simulink model "Receiver_UnderTest_Float"  (R2017b)
settings: Solver=FixedStepDiscrete  StartTime=0.0  StopTime=0.052263  RelTol=1e-3
InitFcn:
  | modelSettingsFloat
undefined symbols (not defined in the file or in its folder): crcDecodeLag, magnitude, numTrainingSamples, RadioSampleRate, samplesPerSymbol, VibertiTracebackLength, xPreambleSeq
libraries: simulink x15, hdlsllib x2, commdigbbndpm3 x2, commsource2 x1, commcrc2 x1, dspstat3 x1, dspsigops x1, commseqgen3 x1, commsequence2 x1, commcnvcod2 x1, commutil2 x1, commfilt2 x1
(part 1 of 2)
settings Model: DataTypeOverride=Off  MinMaxOverflowLogging=MinMaxAndOverflow  FPTRunName=NoOverride  Creator=tcollins  LastModifiedBy=tcollins
settings DataIOCC: SaveOutput=off  SaveTime=off
settings OptimizationCC: BlockReduction=off  ConditionallyExecuteInputs=off  DefaultParameterBehavior=Inlined
settings DebuggingCC: AlgebraicLoopMsg=error  SingleTaskRateTransMsg=error
settings HardwareCC: ProdBitPerPointer=32  ProdBitPerSizeT=32  ProdBitPerPtrDiffT=32  ProdLargestAtomicFloat=None  ProdIntDivRoundTo=Undefined  ProdEndianess=Unspecified  ProdWordSize=32  ProdHWDeviceType=ASIC/FPGA->ASIC/FPGA  ProdEqTarget=off
settings CodeAppCC: StateflowObjectComments=on
settings SimscapeCC: SimscapeNormalizeSystem=off

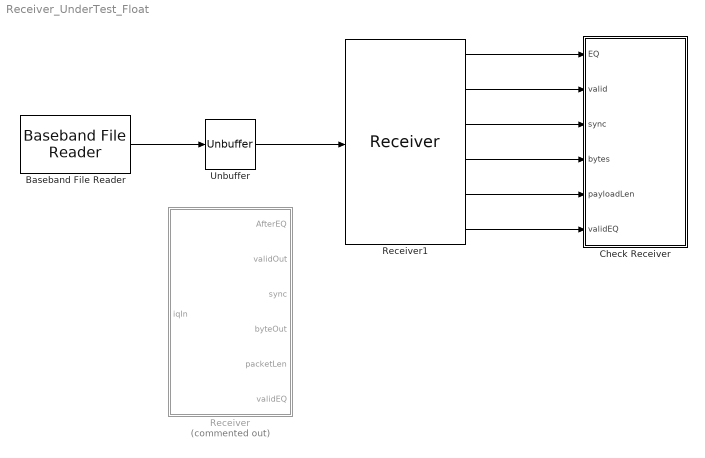
== system Receiver_UnderTest_Float ==
  Baseband File Reader : commsource2/Baseband File Reader  Filename=PlutoCaptureQPSK.bb  InheritSampleTimeFromFile=off  SampleTime=100000/(RadioSampleRate)  SamplesPerFrame=100000  CyclicRepetition=off  FileEndOutputPort=off  SimulateUsing=Interpreted execution
      settings: SourceProductName=Communications System Toolbox  SourceProductBaseCode=CM
  Check Receiver : Subsystem
  Receiver : Subsystem  Commented=on
  Receiver1 : RxFloatingPointLibrary/Receiver
  Unbuffer : Unbuffer
  wires:
  Baseband File Reader/1 -> Unbuffer/1
  Unbuffer/1 -> Receiver1/1
  Receiver1/1 -> Check Receiver/1(EQ)
  Receiver1/2 -> Check Receiver/2(valid)
  Receiver1/3 -> Check Receiver/3(sync)
  Receiver1/4 -> Check Receiver/4(bytes)
  Receiver1/5 -> Check Receiver/5(payloadLen)
  Receiver1/6 -> Check Receiver/6(validEQ)

== system Receiver_UnderTest_Float/Check Receiver ==
  EQ : Inport
  valid : Inport  Port=2
  sync : Inport  Port=3
  bytes : Inport  Port=4
  payloadLen : Inport  Port=5
  validEQ : Inport  Port=6
  Constellation Diagram : Subsystem
  DMA Capture : MATLAB Function  Commented=on  TreatAsAtomicUnit=on
  DMA Capture1 : MATLAB Function  TreatAsAtomicUnit=on
  To Workspace1 : ToWorkspace  VariableName=packetsFound  SaveFormat=Timeseries  SampleTime=-1
  To Workspace2 : ToWorkspace  VariableName=crcChecks  SaveFormat=Timeseries  SampleTime=-1
  To Workspace3 : ToWorkspace  VariableName=failures  SaveFormat=Timeseries  SampleTime=-1
  wires:
  EQ/1 -> Constellation Diagram/1(In1)
  sync/1 -> DMA Capture1/3(sync)
  validEQ/1 -> Constellation Diagram/Enable
  valid/1 -> DMA Capture1/2(validOut)
  bytes/1 -> DMA Capture1/1(bytes)
  payloadLen/1 -> DMA Capture1/4(payloadLen)
  DMA Capture1/2(crc) -> To Workspace2/1
  DMA Capture1/1(pf) -> To Workspace1/1
  DMA Capture1/3(failures) -> To Workspace3/1

== system Receiver_UnderTest_Float/Receiver ==
  iqIn : Inport
  CRC Check and DMA Pack : Subsystem
  Constellation Diagram : Subsystem
  Frame Recover : Subsystem
  Gardner Timing Recovery : Subsystem
  Raised Cosine Receive Filter : commfilt2/Raised Cosine Receive Filter  filtType=Square root  R=0.5  filtSpan=8  N=4  downFactor=1  downOffset=0  filterGain=1  RateOptions=Allow multirate processing  framing=Mute  checkCoeff=off  variableName=rcRxFilt  currentFiltSpan=8  D=(8)/2  inputOffset=0  sampMode=Mute  saveAsFlag=0  rateMode=Downsampling  checkGain=Normalized  launchFVT=on  roundingMode=Floor  overflowMode=off  coeffDataTypeStr=Inherit: Same word length as input  coeffMin=[]  coeffMax=[]  coeffLastDataTypeStr=Inherit: Same word length as input  accumDataTypeStr=Inherit: Same as product output  accumLastDataTypeStr=Inherit: Same as product output  outputDataTypeStr=Inherit: Same as accumulator  outputMin=[]  outputMax=[]  outputLastDataTypeStr=Inherit: Same as accumulator
  AfterEQ : Outport
  validOut : Outport  Port=2
  sync : Outport  Port=3
  byteOut : Outport  Port=4
  packetLen : Outport  Port=5
  validEQ : Outport  Port=6
  wires:
  Frame Recover/2(validOut) -> CRC Check and DMA Pack/1(validIn), validEQ/1
  CRC Check and DMA Pack/4(payloadLenOut) -> packetLen/1
  CRC Check and DMA Pack/3(sync) -> sync/1
  CRC Check and DMA Pack/1(byteOut) -> byteOut/1
  CRC Check and DMA Pack/2(validOut) -> validOut/1
  Frame Recover/6(packetLen) -> CRC Check and DMA Pack/5(payloadLen)
  Frame Recover/3(data) -> CRC Check and DMA Pack/2(bits)
  Frame Recover/5(frameEnd) -> CRC Check and DMA Pack/4(endCRC)
  Frame Recover/4(frameStart) -> CRC Check and DMA Pack/3(startData)
  Frame Recover/1(AfterEQ) -> AfterEQ/1
  iqIn/1 -> Raised Cosine Receive Filter/1
  Raised Cosine Receive Filter/1 -> Gardner Timing Recovery/1(dataIn)
  Gardner Timing Recovery/2(strobe) -> Frame Recover/Enable, Frame Recover/2(validIn), Constellation Diagram/Enable
  Gardner Timing Recovery/1(dataOut) -> Frame Recover/1(dataIn), Constellation Diagram/1(In1)

== system Receiver_UnderTest_Float/Check Receiver/Constellation Diagram ==
  In1 : Inport
  Enable : EnablePort
  Terminator : Terminator
  wires:
  In1/1 -> Terminator/1

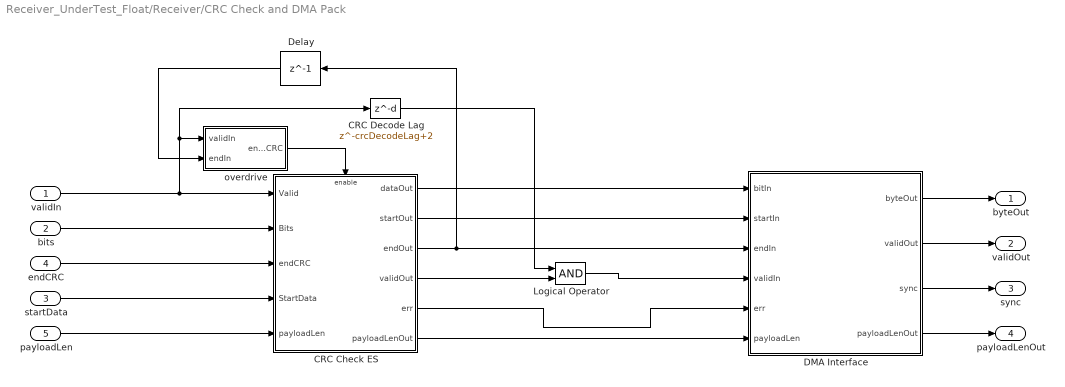
== system Receiver_UnderTest_Float/Receiver/CRC Check and DMA Pack ==
  validIn : Inport
  bits : Inport  Port=2
  startData : Inport  Port=3
  endCRC : Inport  Port=4
  payloadLen : Inport  Port=5
  CRC Check ES : Subsystem
  CRC Decode Lag : Delay  DelayLength=crcDecodeLag+2
  DMA Interface : Subsystem
  Delay : Delay  DelayLength=1
  Logical Operator : Logic  AllPortsSameDT=off  OutDataTypeStr=boolean
  overdrive : MATLAB Function  TreatAsAtomicUnit=on
  byteOut : Outport
  validOut : Outport  Port=2
  sync : Outport  Port=3
  payloadLenOut : Outport  Port=4
  wires:
  overdrive/1(enableCRC) -> CRC Check ES/Enable
  DMA Interface/4(payloadLenOut) -> payloadLenOut/1
  Delay/1 -> overdrive/2(endIn)
  validIn/1 -> overdrive/1(validIn), CRC Decode Lag/1, CRC Check ES/1(Valid)
  CRC Check ES/4(validOut) -> Logical Operator/2
  CRC Decode Lag/1 -> Logical Operator/1
  CRC Check ES/6(payloadLenOut) -> DMA Interface/6(payloadLen)
  CRC Check ES/5(err) -> DMA Interface/5(err)
  Logical Operator/1 -> DMA Interface/4(validIn)
  CRC Check ES/3(endOut) -> Delay/1, DMA Interface/3(endIn)
  CRC Check ES/2(startOut) -> DMA Interface/2(startIn)
  CRC Check ES/1(dataOut) -> DMA Interface/1(bitIn)
  endCRC/1 -> CRC Check ES/3(endCRC)
  startData/1 -> CRC Check ES/4(StartData)
  payloadLen/1 -> CRC Check ES/5(payloadLen)
  DMA Interface/3(sync) -> sync/1
  bits/1 -> CRC Check ES/2(Bits)
  DMA Interface/1(byteOut) -> byteOut/1
  DMA Interface/2(validOut) -> validOut/1

== system Receiver_UnderTest_Float/Receiver/Constellation Diagram ==
  In1 : Inport
  Enable : EnablePort
  wires:
  In1/1 -> ?

== system Receiver_UnderTest_Float/Receiver/Frame Recover ==
  dataIn : Inport
  validIn : Inport  Port=2
  Enable : EnablePort
  Barker Locate : Subsystem  mask{Threshold=1.4}
  Enable Equalizer and Packet Decode (Latch) : MATLAB Function  TreatAsAtomicUnit=on
  Equalization and Demodulation : Subsystem
  Frequency Recovery : Subsystem
  AfterEQ : Outport
  validOut : Outport  Port=2  OutputWhenDisabled=reset  InitialOutput=0
  data : Outport  Port=3
  frameStart : Outport  Port=4
  frameEnd : Outport  Port=5
  packetLen : Outport  Port=6
  wires:
  Equalization and Demodulation/6(frameStart) -> frameStart/1
  Equalization and Demodulation/4(dataOut) -> data/1
  Equalization and Demodulation/1(AfterEQ) -> AfterEQ/1
  Equalization and Demodulation/2(validOut) -> validOut/1
  Equalization and Demodulation/3(crcEnd) -> frameEnd/1
  Enable Equalizer and Packet Decode (Latch)/1(enable) -> Equalization and Demodulation/Enable
  Barker Locate/2(Signal) -> Equalization and Demodulation/2(Data)
  Barker Locate/3(enableOut) -> Enable Equalizer and Packet Decode (Latch)/2(validIn)
  Barker Locate/1(Detector) -> Equalization and Demodulation/1(Trigger), Enable Equalizer and Packet Decode (Latch)/1(start)
  Equalization and Demodulation/5(packLen) -> packetLen/1
  Frequency Recovery/1(dataOut) -> Barker Locate/1(In1)
  Frequency Recovery/2(validOut) -> Barker Locate/2(enableIn)
  dataIn/1 -> Frequency Recovery/1(dataIn)
  validIn/1 -> Frequency Recovery/2(validIn)

== system Receiver_UnderTest_Float/Receiver/Gardner Timing Recovery ==
  dataIn : Inport
  Delay : Delay  DelayLength=1
  Delay1 : Delay  DelayLength=1
  Gardner TED Blocks : Subsystem
  InterpControl_Blocks1 : Subsystem
  Interpolator : Subsystem
  LoopFilter : Subsystem  mask{zeta=sqrt(2), BnTs=0.01, Kp=2.7}
      mask prompts: zeta "DampingFactor"; BnTs "NormalizedLoopBandwidth"; Kp "DetectionGain"
      mask init:
      | K0 = -1;
      | SPS = 4;
      | theta = BnTs/SPS/(zeta + 0.25/zeta);
      | d  = (1 + 2*zeta*theta + theta^2) * K0 * Kp;
      | ProportionalGain = (4*zeta*theta) /d;
      | IntegratorGain   = (4*theta*theta)/d;
  dataOut : Outport  InitialOutput=0
  strobe : Outport  Port=2  InitialOutput=false
  wires:
  dataIn/1 -> Interpolator/1(In1)
  LoopFilter/1(v) -> InterpControl_Blocks1/1(e)
  InterpControl_Blocks1/2(mu) -> Delay/1
  InterpControl_Blocks1/1(strobe) -> Delay1/1
  Gardner TED Blocks/1(e) -> LoopFilter/1(e)
  Interpolator/1(Out1) -> dataOut/1, Gardner TED Blocks/1(data)
  Delay/1 -> Interpolator/2(mu)
  Delay1/1 -> strobe/1, Gardner TED Blocks/2(strobe)

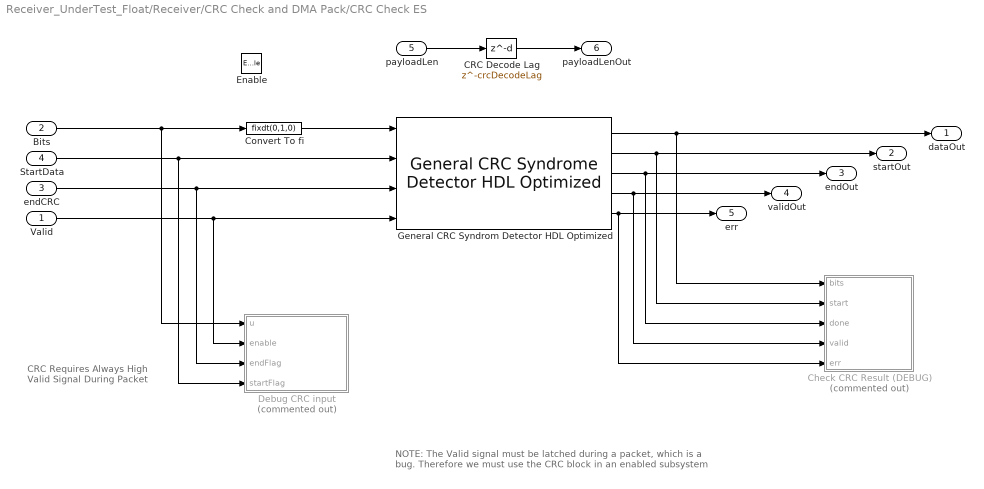
== system Receiver_UnderTest_Float/Receiver/CRC Check and DMA Pack/CRC Check ES ==
  note: CRC Requires
      | Always High
      | Valid Signal During
      | Packet
  note: NOTE:
      | 	The Valid signal must be latched during a packet, which is
      | 	a bug.  Therefore we must use the CRC block in an enabled
      | 	subsystem
  Valid : Inport
  Bits : Inport  Port=2
  endCRC : Inport  Port=3
  StartData : Inport  Port=4
  payloadLen : Inport  Port=5
  Enable : EnablePort
  CRC Decode Lag : Delay  DelayLength=crcDecodeLag
  Check CRC Result (DEBUG) : MATLAB Function  Commented=on  TreatAsAtomicUnit=on
  Convert To fi : DataTypeConversion  OutDataTypeStr=fixdt(0,1,0)  SaturateOnIntegerOverflow=on
  Debug CRC input : MATLAB Function  Commented=on  TreatAsAtomicUnit=on
  General CRC Syndrom Detector HDL Optimized : commcrc2/General CRC Syndrome Detector HDL Optimized  Polynomial=crc32Poly  InitialState=0  DirectMethod=off  ReflectInput=off  ReflectCRCChecksum=off  FinalXORValue=0  SimulateUsing=Code generation
      settings: SourceProductName=Communications System Toolbox  SourceProductBaseCode=CM
  dataOut : Outport  InitialOutput=0
  startOut : Outport  Port=2  InitialOutput=0
  endOut : Outport  Port=3  InitialOutput=0
  validOut : Outport  Port=4  InitialOutput=0
  err : Outport  Port=5  InitialOutput=0
  payloadLenOut : Outport  Port=6  InitialOutput=0
  wires:
  Valid/1 -> Debug CRC input/2(enable), General CRC Syndrom Detector HDL Optimized/4
  endCRC/1 -> General CRC Syndrom Detector HDL Optimized/3, Debug CRC input/3(endFlag)
  StartData/1 -> General CRC Syndrom Detector HDL Optimized/2, Debug CRC input/4(startFlag)
  CRC Decode Lag/1 -> payloadLenOut/1
  payloadLen/1 -> CRC Decode Lag/1
  Convert To fi/1 -> General CRC Syndrom Detector HDL Optimized/1
  General CRC Syndrom Detector HDL Optimized/2 -> startOut/1, Check CRC Result (DEBUG)/2(start)
  General CRC Syndrom Detector HDL Optimized/5 -> err/1, Check CRC Result (DEBUG)/5(err)
  General CRC Syndrom Detector HDL Optimized/4 -> validOut/1, Check CRC Result (DEBUG)/4(valid)
  General CRC Syndrom Detector HDL Optimized/3 -> endOut/1, Check CRC Result (DEBUG)/3(done)
  General CRC Syndrom Detector HDL Optimized/1 -> dataOut/1, Check CRC Result (DEBUG)/1(bits)
  Bits/1 -> Debug CRC input/1(u), Convert To fi/1

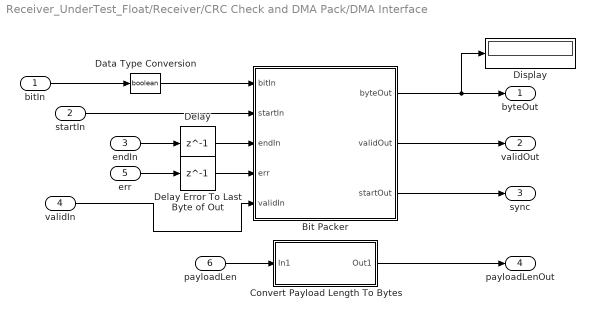
== system Receiver_UnderTest_Float/Receiver/CRC Check and DMA Pack/DMA Interface ==
  bitIn : Inport
  startIn : Inport  Port=2
  endIn : Inport  Port=3
  validIn : Inport  Port=4
  err : Inport  Port=5
  payloadLen : Inport  Port=6
  Bit Packer : MATLAB Function  TreatAsAtomicUnit=on
  Convert Payload Length To Bytes : Subsystem
  Data Type Conversion : DataTypeConversion  OutDataTypeStr=boolean
  Delay : Delay  DelayLength=1
  Delay Error To Last Byte of Out : Delay  DelayLength=1
  Display : Display
  byteOut : Outport
  validOut : Outport  Port=2
  sync : Outport  Port=3
  payloadLenOut : Outport  Port=4
  wires:
  Convert Payload Length To Bytes/1(Out1) -> payloadLenOut/1
  payloadLen/1 -> Convert Payload Length To Bytes/1(In1)
  Data Type Conversion/1 -> Bit Packer/1(bitIn)
  startIn/1 -> Bit Packer/2(startIn)
  endIn/1 -> Delay/1
  validIn/1 -> Bit Packer/5(validIn)
  err/1 -> Delay Error To Last Byte of Out/1
  Bit Packer/1(byteOut) -> byteOut/1, Display/1
  Bit Packer/3(startOut) -> sync/1
  Bit Packer/2(validOut) -> validOut/1
  Delay Error To Last Byte of Out/1 -> Bit Packer/4(err)
  Delay/1 -> Bit Packer/3(endIn)
  bitIn/1 -> Data Type Conversion/1

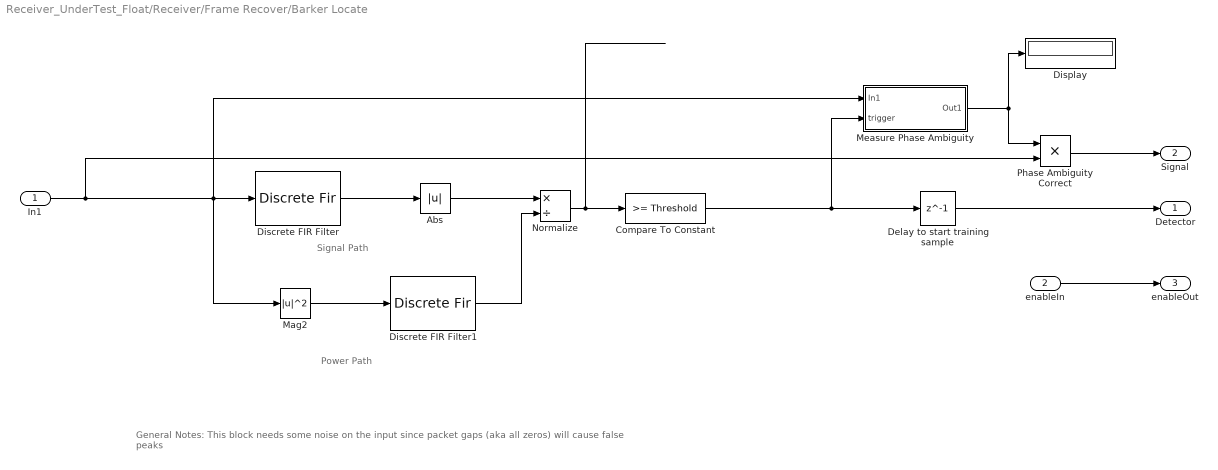
== system Receiver_UnderTest_Float/Receiver/Frame Recover/Barker Locate ==
  note: Signal Path
  note: Power Path
  note: General Notes:
      | This block needs some noise on the input since packet gaps (aka all zeros) will cause false peaks
  In1 : Inport
  enableIn : Inport  Port=2
  Abs : Abs
  Compare To Constant : simulink/Logic and Bit Operations/Compare To Constant  relop=>=  const=Threshold  OutDataTypeStr=boolean
  "Delay to start training sample " : Delay  DelayLength=1
  Discrete FIR Filter : DiscreteFir  Coefficients=xPreambleSeq(end:-1:1).'  AccumDataTypeStr=Inherit: Same as product output  OutDataTypeStr=Inherit: Same as input
  Discrete FIR Filter1 : DiscreteFir  Coefficients=ones(1,length(xPreambleSeq)*1)/1  InitialStates=1  AccumDataTypeStr=Inherit: Same as product output  OutDataTypeStr=Inherit: Same as input
  Display : Display
  Mag2 : Math  Operator=magnitude^2  SaturateOnIntegerOverflow=on
  Measure Phase Ambiguity : Subsystem
  Normalize : Product  Inputs=*/
  Phase Ambiguity Correct : Product
  Detector : Outport
  Signal : Outport  Port=2
  enableOut : Outport  Port=3
  wires:
  In1/1 -> Measure Phase Ambiguity/1(In1), Discrete FIR Filter/1, Mag2/1, Phase Ambiguity Correct/2
  "Delay to start training sample "/1 -> Detector/1
  enableIn/1 -> enableOut/1
  Mag2/1 -> Discrete FIR Filter1/1
  Discrete FIR Filter1/1 -> Normalize/2
  Measure Phase Ambiguity/1(Out1) -> Phase Ambiguity Correct/1, Display/1
  Phase Ambiguity Correct/1 -> Signal/1
  Normalize/1 -> Compare To Constant/1
  Compare To Constant/1 -> Measure Phase Ambiguity/2(trigger), "Delay to start training sample "/1
  Abs/1 -> Normalize/1
  Discrete FIR Filter/1 -> Abs/1

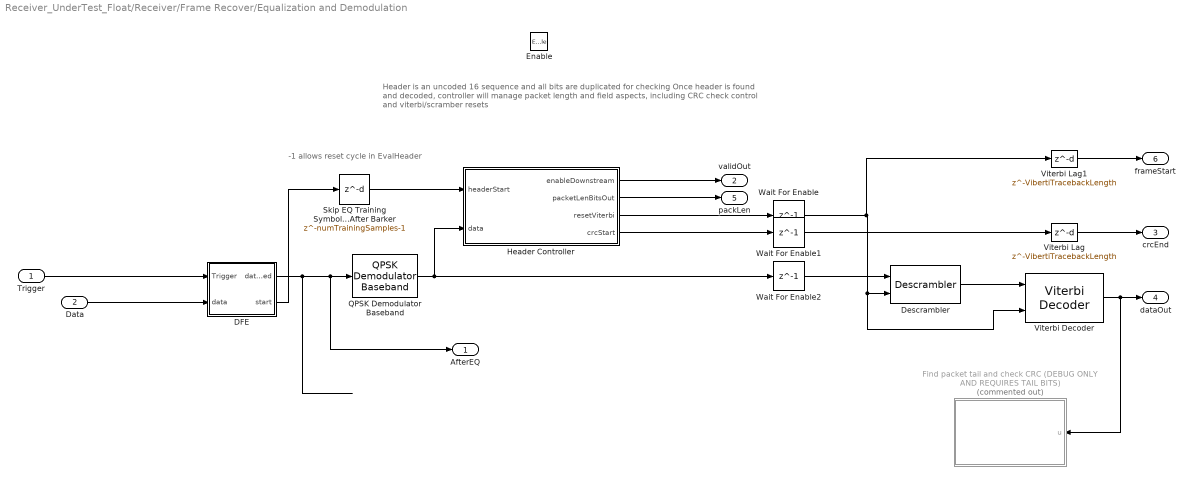
== system Receiver_UnderTest_Float/Receiver/Frame Recover/Equalization and Demodulation ==
  note: Header is an uncoded 16 sequence and all bits are duplicated for checking
      |
      | Once header is found and decoded, controller will manage packet length and field aspects,
      | including CRC check control and viterbi/scramber resets
  note: -1 allows reset cycle in EvalHeader
  Trigger : Inport
  Data : Inport  Port=2
  Enable : EnablePort
  DFE : Subsystem
  Descrambler : commsequence2/Descrambler  M=2  poly='1 + z^-1 + z^-3 + z^-5+ z^-7'  iniStaSource=Dialog Parameter  ini_sta=[0 1 0 0 0 1 0]  resetViaPort=on
      settings: SourceProductName=Communications System Toolbox  SourceProductBaseCode=CM
  Find packet tail and check CRC (DEBUG ONLY AND REQUIRES TAIL BITS) : MATLAB Function  Commented=on  TreatAsAtomicUnit=on
  Header Controller : MATLAB Function  TreatAsAtomicUnit=on
  QPSK Demodulator Baseband : commdigbbndpm3/QPSK Demodulator Baseband  OutType=Bit  DecType=Hard decision  VarSource=Dialog  Variance=1  Dec=Binary  Ph=pi/4  outDtype1=boolean  outDtype2=Inherit via internal rule  derotateFactorWordLen=16  derotateFactorDataTypeStr=Inherit: Same word length as input  derotateFactorLastDataTypeStr=Inherit: Same word length as input
  Skip EQ Training Symbols After Barker : Delay  DelayLength=numTrainingSamples-1
  Viterbi Decoder : commcnvcod2/Viterbi Decoder  trellis=poly2trellis(7, [171 133])  isPunctured=off  punctureVector=[1; 1; 0; 1; 0; 1]  erasures=off  dectype=Hard decision  nsdecb=4  runSigValErrCheck=off  tbdepth=VibertiTracebackLength  opmode=Continuous  reset=on  delayedResetAction=on  smWordLength=16  outDataType=boolean
      settings: SourceProductName=Communications System Toolbox  SourceProductBaseCode=CM
  Viterbi Lag : Delay  DelayLength=VibertiTracebackLength
  Viterbi Lag1 : Delay  DelayLength=VibertiTracebackLength
  Wait For Enable : Delay  DelayLength=1
  Wait For Enable1 : Delay  DelayLength=1
  Wait For Enable2 : Delay  DelayLength=1
  AfterEQ : Outport  InitialOutput=0
  validOut : Outport  Port=2  InitialOutput=0
  crcEnd : Outport  Port=3  InitialOutput=0
  dataOut : Outport  Port=4  InitialOutput=0
  packLen : Outport  Port=5  InitialOutput=0
  frameStart : Outport  Port=6  InitialOutput=0
  wires:
  Viterbi Lag1/1 -> frameStart/1
  Viterbi Lag/1 -> crcEnd/1
  Viterbi Decoder/1 -> dataOut/1, Find packet tail and check CRC (DEBUG ONLY AND REQUIRES TAIL BITS)/1(u)
  DFE/2(start) -> Skip EQ Training Symbols After Barker/1
  Data/1 -> DFE/2(data)
  Trigger/1 -> DFE/1(Trigger)
  Descrambler/1 -> Viterbi Decoder/1
  Wait For Enable2/1 -> Descrambler/1
  Wait For Enable1/1 -> Viterbi Lag/1
  Wait For Enable/1 -> Descrambler/2, Viterbi Decoder/2, Viterbi Lag1/1
  Header Controller/2(packetLenBitsOut) -> packLen/1
  Header Controller/3(resetViterbi) -> Wait For Enable/1
  Header Controller/4(crcStart) -> Wait For Enable1/1
  Header Controller/1(enableDownstream) -> validOut/1
  QPSK Demodulator Baseband/1 -> Wait For Enable2/1, Header Controller/2(data)
  DFE/1(dataEQed) -> QPSK Demodulator Baseband/1, AfterEQ/1
  Skip EQ Training Symbols After Barker/1 -> Header Controller/1(headerStart)

== system Receiver_UnderTest_Float/Receiver/Frame Recover/Frequency Recovery ==
  note: Pull in range (Hz) = 2*pi*sqrt(2)*DampingFactor*NormLoopBandwidth*SampleRate
  note: Frequency Lock Delay = SampleRate*4*NormalizedPullInRange^2)/ (SampleRate*NormLoopBandwidth)^3;
  note: Max Phase Lock Delay= 1.3/(NormLoopBandwidth*SampleRate)
  dataIn : Inport
  validIn : Inport  Port=2
  Delay : Delay  DelayLength=1
  Loop Filter : Subsystem  mask{BnTs=0.1, zeta=3*1/sqrt(2), N=1}
      mask prompts: BnTs "Normalized Loop Bandwidth"; zeta "Damping Factor"; N "Number of Samples/Symbol"
      mask init:
      | % See C.57 to C.61 in Michael Rice's "Digital Communications 
      | % - A Discrete-Time Approach" for details
      | 
      | %theta = BnTs/(zeta+0.25/zeta);  %0.0385
      | %d = 1 + 2*zeta*theta + theta*theta; %1.1938
      | %K1 = zeta*theta/d; %0.0805
      | %K2 = theta*theta/(d*2); %6.1958e-04
      | 
      | %%
      | DampingFactor = zeta;
      | samplesPerSymbol = N;
      | NormalizedLoopBandwidth = BnTs;
      | %
      | PhaseRecoveryLoopBandwidth = NormalizedLoopBandwidth*samplesPerSymbol;
      |  
      | PhaseRecoveryGain = samplesPerSymbol;
      |  
      | PhaseErrorDetectorGain = 1;
      | 
      | 
      | theta = PhaseRecoveryLoopBandwidth/...
      |     ((DampingFactor + 0.25/DampingFactor)*samplesPerSymbol);
      |  
      | d = 1 + 2*DampingFactor*theta + theta*theta;
      |  
      | % K1
      | K1 = (4*DampingFactor*theta/d)/...
      |     (PhaseErrorDetectorGain*PhaseRecoveryGain);
      | % K2
      | K2 = (4/samplesPerSymbol*theta*theta/d)/...
      |     (PhaseErrorDetectorGain*PhaseRecoveryGain);
      mask Display: disp('Loop Filter')
  PED : MATLAB Function  TreatAsAtomicUnit=on
  Phase Shift FP : Subsystem
  dataOut : Outport
  validOut : Outport  Port=2
  wires:
  validIn/1 -> validOut/1
  Phase Shift FP/1(Out1) -> Delay/1
  dataIn/1 -> Phase Shift FP/1(In1)
  Loop Filter/1(v) -> Phase Shift FP/2(Phi)
  PED/1(e) -> Loop Filter/1(e)
  Delay/1 -> PED/1(In), dataOut/1

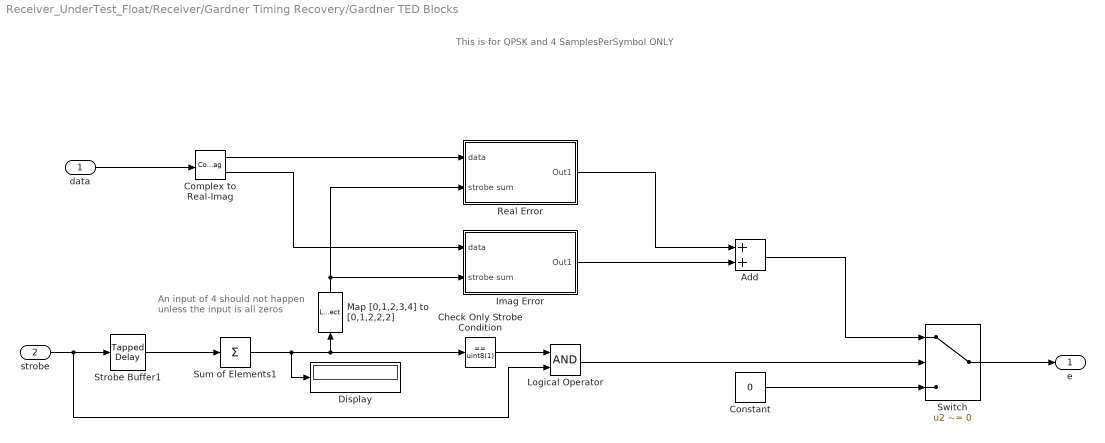
== system Receiver_UnderTest_Float/Receiver/Gardner Timing Recovery/Gardner TED Blocks ==
  note: This is for QPSK and 4 SamplesPerSymbol ONLY
  note: An input of 4 should not
      | happen unless the input is all zeros
  data : Inport
  strobe : Inport  Port=2
  Add : Sum  OutDataTypeStr=Inherit: Inherit via back propagation
  Check Only Strobe Condition : simulink/Logic and Bit Operations/Compare To Constant  relop===  const=uint8(1)  OutDataTypeStr=boolean
  Complex to Real-Imag : ComplexToRealImag
  Constant : Constant  Value=0  SampleTime=-1
  Display : Display
  Imag Error : Subsystem
  Logical Operator : Logic  AllPortsSameDT=off  OutDataTypeStr=boolean
  Map [0,1,2,3,4] to [0,1,2,2,2] : LookupNDDirect  NumberOfTableDimensions=1  Table=[0 1 2 2 2]  DiagnosticForOutOfRangeInput=Error  TableDataTypeStr=uint8
  Real Error : Subsystem
  Strobe Buffer1 : simulink/Discrete/Tapped Delay  vinit=0.0  samptime=-1  NumDelays=samplesPerSymbol-1  DelayOrder=Oldest  includeCurrent=on
  Sum of Elements1 : Sum  Inputs=+  OutDataTypeStr=int8
  Switch : Switch  Criteria=u2 ~= 0  OutDataTypeStr=Inherit: Inherit via back propagation  SaturateOnIntegerOverflow=on
  e : Outport
  wires:
  Logical Operator/1 -> Switch/2
  Add/1 -> Switch/1
  Imag Error/1(Out1) -> Add/2
  Real Error/1(Out1) -> Add/1
  Strobe Buffer1/1 -> Sum of Elements1/1
  Map [0,1,2,3,4] to [0,1,2,2,2]/1 -> Real Error/2(strobe sum), Imag Error/2(strobe sum)
  data/1 -> Complex to Real-Imag/1
  Complex to Real-Imag/1 -> Real Error/1(data)
  Constant/1 -> Switch/3
  Check Only Strobe Condition/1 -> Logical Operator/1
  Sum of Elements1/1 -> Map [0,1,2,3,4] to [0,1,2,2,2]/1, Check Only Strobe Condition/1, Display/1
  Complex to Real-Imag/2 -> Imag Error/1(data)
  strobe/1 -> Logical Operator/2, Strobe Buffer1/1
  Switch/1 -> e/1

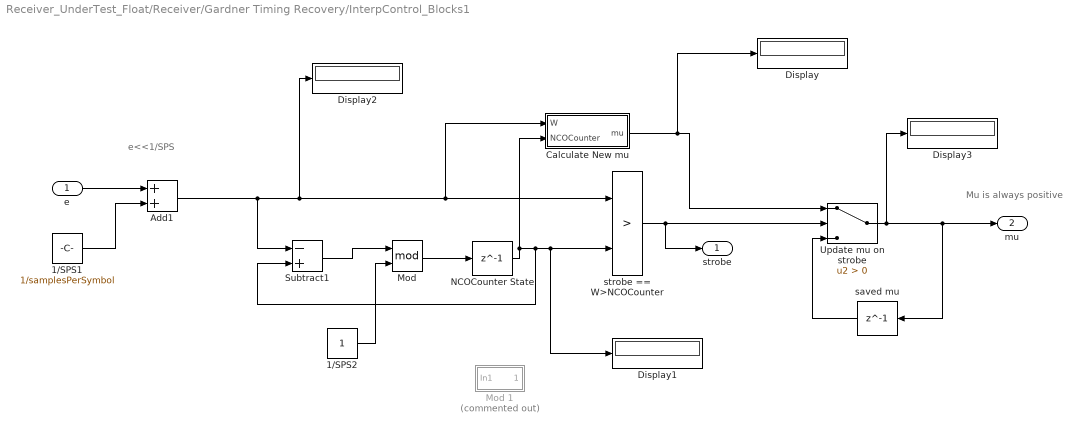
== system Receiver_UnderTest_Float/Receiver/Gardner Timing Recovery/InterpControl_Blocks1 ==
  note: Mu is always positive
  note: e<<1/SPS
  e : Inport
  1/SPS1 : Constant  Value=1/samplesPerSymbol  SampleTime=-1
  1/SPS2 : Constant  SampleTime=-1
  Add1 : Sum  OutDataTypeStr=Inherit: Inherit via back propagation
  Calculate New mu : Subsystem
  Display{,1..3} (4 alike) : Display
  Mod : Math  Operator=mod  SaturateOnIntegerOverflow=on
  Mod 1 : Subsystem  Commented=on
  NCOCounter State : Delay  DelayLength=1  InitialCondition=0
  Subtract1 : Sum  Inputs=-+  OutDataTypeStr=Inherit: Same as first input
  Update mu on strobe : Switch  Criteria=u2 > Threshold
  saved mu : Delay  DelayLength=1
  strobe == W>NCOCounter : RelationalOperator  Operator=>  OutDataTypeStr=boolean  RndMeth=Nearest
  strobe : Outport
  mu : Outport  Port=2
  wires:
  1/SPS2/1 -> Mod/2
  Add1/1 -> Subtract1/1, Display2/1, strobe == W>NCOCounter/1, Calculate New mu/1(W)
  1/SPS1/1 -> Add1/2
  Mod/1 -> NCOCounter State/1
  Subtract1/1 -> Mod/1
  NCOCounter State/1 -> Calculate New mu/2(NCOCounter), strobe == W>NCOCounter/2, Display1/1, Subtract1/2
  e/1 -> Add1/1
  Calculate New mu/1(mu) -> Update mu on strobe/1, Display/1
  saved mu/1 -> Update mu on strobe/3
  Update mu on strobe/1 -> saved mu/1, mu/1, Display3/1
  strobe == W>NCOCounter/1 -> strobe/1, Update mu on strobe/2

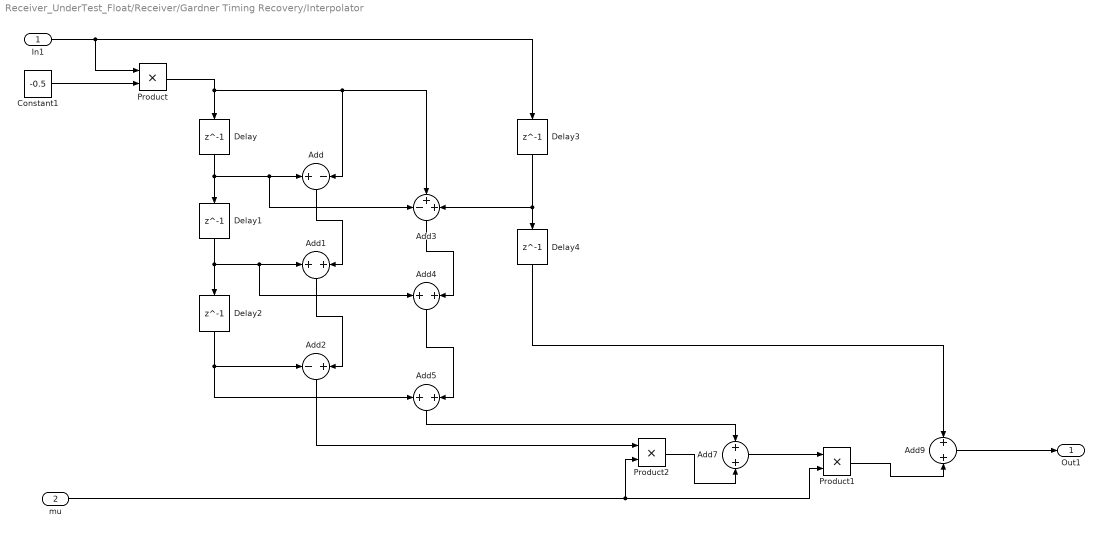
== system Receiver_UnderTest_Float/Receiver/Gardner Timing Recovery/Interpolator ==
  In1 : Inport
  mu : Inport  Port=2
  Add : Sum  Inputs=+-  OutDataTypeStr=Inherit: Same as first input
  Add{1,4..5,7,9} (5 alike) : Sum
  Add2 : Sum  Inputs=-+
  Add3 : Sum  Inputs=-++
  Constant1 : Constant  Value=-0.5  OutDataTypeStr=double  SampleTime=-1
  Delay{,1..4} (5 alike) : Delay  DelayLength=1
  Product : Product  OutDataTypeStr=double
  Product1 : Product
  Product2 : Product
  Out1 : Outport
  wires:
  Add9/1 -> Out1/1
  mu/1 -> Product2/2, Product1/2
  Add7/1 -> Product1/1
  Delay4/1 -> Add9/1
  Add2/1 -> Product2/1
  Add5/1 -> Add7/1
  Constant1/1 -> Product/2
  Product1/1 -> Add9/2
  Delay3/1 -> Add3/3, Delay4/1
  Product2/1 -> Add7/2
  Add4/1 -> Add5/2
  Add3/1 -> Add4/2
  Add1/1 -> Add2/2
  Delay2/1 -> Add2/1, Add5/1
  Add/1 -> Add1/2
  Delay1/1 -> Delay2/1, Add1/1, Add4/1
  Delay/1 -> Delay1/1, Add/1, Add3/1
  Product/1 -> Delay/1, Add/2, Add3/2
  In1/1 -> Product/1, Delay3/1

== system Receiver_UnderTest_Float/Receiver/Gardner Timing Recovery/LoopFilter ==
  e : Inport
  Add : Sum
  Add1 : Sum
  Delay : Delay  DelayLength=1
  Delay1 : Delay  DelayLength=1
  Intergrator Gain : Gain  Gain=IntegratorGain
  Proportional Gain : Gain  Gain=ProportionalGain
  v : Outport
  wires:
  Proportional Gain/1 -> Add1/2
  Add1/1 -> v/1
  Delay1/1 -> Add/2
  Delay/1 -> Add/1
  Intergrator Gain/1 -> Delay/1
  e/1 -> Intergrator Gain/1, Proportional Gain/1
  Add/1 -> Delay1/1, Add1/1

== system Receiver_UnderTest_Float/Receiver/CRC Check and DMA Pack/DMA Interface/Convert Payload Length To Bytes ==
  In1 : Inport
  Constant : Constant  Value=uint16(32-1)  SampleTime=-1
  Convert To Bytes From Bits : ArithShift  BitShiftNumber=3  BitShiftDirection=Right
  Convert To Uncoded : ArithShift  BitShiftNumber=1  BitShiftDirection=Right
  Data Type Conversion : DataTypeConversion  OutDataTypeStr=int16
  Remove CRC Length : Sum  Inputs=+-  AccumDataTypeStr=uint16
  Out1 : Outport
  wires:
  Data Type Conversion/1 -> Out1/1
  Constant/1 -> Remove CRC Length/2
  Convert To Bytes From Bits/1 -> Data Type Conversion/1
  Convert To Uncoded/1 -> Remove CRC Length/1
  Remove CRC Length/1 -> Convert To Bytes From Bits/1
  In1/1 -> Convert To Uncoded/1

== system Receiver_UnderTest_Float/Receiver/Frame Recover/Barker Locate/Measure Phase Ambiguity ==
  In1 : Inport
  trigger : Inport  Port=2
  Discrete FIR Filter1 : DiscreteFir  Coefficients=exp(-j*pi/2).*xPreambleSeq(end:-1:1).'  InputProcessing=Columns as channels (frame based)  AccumDataTypeStr=Inherit: Same as product output  OutDataTypeStr=Inherit: Same as input
  Discrete FIR Filter2 : DiscreteFir  Coefficients=xPreambleSeq(end:-1:1).'  InputProcessing=Columns as channels (frame based)  AccumDataTypeStr=Inherit: Same as product output  OutDataTypeStr=Inherit: Same as input
  Discrete FIR Filter3 : DiscreteFir  Coefficients=exp(-j*pi).*xPreambleSeq(end:-1:1).'  InputProcessing=Columns as channels (frame based)  AccumDataTypeStr=Inherit: Same as product output  OutDataTypeStr=Inherit: Same as input
  Discrete FIR Filter4 : DiscreteFir  Coefficients=exp(-j*pi*3/2).*xPreambleSeq(end:-1:1).'  InputProcessing=Columns as channels (frame based)  AccumDataTypeStr=Inherit: Same as product output  OutDataTypeStr=Inherit: Same as input
  Find Max and Set Output Shift : Subsystem
  Get Index of max : MATLAB Function  Commented=on  TreatAsAtomicUnit=on
  Out1 : Outport
  wires:
  Find Max and Set Output Shift/1(Out1) -> Out1/1
  trigger/1 -> Get Index of max/5(trigger), Find Max and Set Output Shift/5(Trigger)
  Discrete FIR Filter4/1 -> Get Index of max/4(pi34), Find Max and Set Output Shift/4(In5)
  Discrete FIR Filter3/1 -> Get Index of max/3(pi2), Find Max and Set Output Shift/3(In4)
  Discrete FIR Filter1/1 -> Get Index of max/2(pi4), Find Max and Set Output Shift/2(In2)
  Discrete FIR Filter2/1 -> Get Index of max/1(noShift), Find Max and Set Output Shift/1(In1)
  In1/1 -> Discrete FIR Filter2/1, Discrete FIR Filter1/1, Discrete FIR Filter3/1, Discrete FIR Filter4/1

== system Receiver_UnderTest_Float/Receiver/Frame Recover/Equalization and Demodulation/DFE ==
  note: Generate training sequence when barker is found
  Trigger : Inport
  data : Inport  Port=2  PortDimensions=1
  DFE1 : Subsystem  mask{numFTaps=5, numBTaps=3, mu=0.01, refTap=2}
      mask prompts: numFTaps "Num Forward Taps"; numBTaps "Num Backward Taps"; mu "Step Size"; refTap "Reference Tap"
  DFE2 : Subsystem  Commented=on  mask{numFTaps=11, numBTaps=3, mu=0.01}
      mask prompts: numFTaps "Num Forward Taps"; numBTaps "Num Backward Taps"; mu "Step Size"
  Delay data so DFE can reset : Delay  DelayLength=1
  Delay ref so DFE can reset : Delay  DelayLength=1
  Equalizer : MATLAB Function  Commented=on  TreatAsAtomicUnit=on
  PN Sequence Generator : commseqgen3/PN Sequence Generator  poly='z^5 + z^3 + z^1 + 1'  ini_sta=[1 1 1 0 0]  outBitMaskSource=Dialog parameter  shift=0  outVarSiz=off  maxOutSizeMode=Dialog parameter  maxOutSize=[10 1]  Ts=-1  sampPerFrame=1  reset=on  bitPackedOutputs=on  outDataType=Smallest unsigned integer  numPackedBits=2  bitPackDataSigned=off  bitPackedOutDType=Smallest integer
      settings: SourceProductName=Communications System Toolbox
  Packeted To Unpacked : Subsystem
  QPSK Modulator Baseband : commdigbbndpm3/QPSK Modulator Baseband  InType=Bit  Enc=Binary  Ph=pi/4  outDtype=double  outWordLen=16  outUDDataType=sfix(16)  outFracLenMode=User-defined  outFracLen=14  outDataTypeStr=double  outLastDataTypeStr=double
  Terminator : Terminator
  dataEQed : Outport
  start : Outport  Port=2
  wires:
  DFE1/3(start) -> start/1
  Delay data so DFE can reset/1 -> DFE1/2(dataIn)
  Trigger/1 -> PN Sequence Generator/1, DFE1/1(reset)
  Delay ref so DFE can reset/1 -> DFE1/3(training)
  DFE1/1(eqOut) -> dataEQed/1
  DFE1/2(err) -> Terminator/1
  QPSK Modulator Baseband/1 -> Delay ref so DFE can reset/1
  Packeted To Unpacked/1(Out1) -> QPSK Modulator Baseband/1
  PN Sequence Generator/1 -> Packeted To Unpacked/1(In1)
  data/1 -> Delay data so DFE can reset/1

== system Receiver_UnderTest_Float/Receiver/Frame Recover/Frequency Recovery/Loop Filter ==
  note: Proportional-plus-Integrator Loop Filter,
      | Infinite DC Response to guarantee convergence
  note: This inflation is necessary
  e : Inport
  Add1 : Sum  RndMeth=Nearest  OutDataTypeStr=Inherit: Same as first input
  Add2 : Sum  OutDataTypeStr=Inherit: Same as first input
  Delay : Delay  DelayLength=1
  Delay3 : Delay  DelayLength=1
  Delay4 : Delay  DelayLength=1
  Gain : Gain  Gain=-1.0
  K1 : Gain  Gain=K2  OutDataTypeStr=Inherit: Same as input
  K2 : Gain  Gain=K1  OutDataTypeStr=Inherit: Same as input
  Sum2 : Sum  OutDataTypeStr=Inherit: Same as first input
  v : Outport
  wires:
  Gain/1 -> v/1
  Add2/1 -> Gain/1, Delay4/1
  Delay4/1 -> Add2/2
  Delay3/1 -> Add2/1
  Sum2/1 -> Delay3/1
  Delay/1 -> Add1/1
  K2/1 -> Add1/2, Delay/1
  e/1 -> K1/1, K2/1
  Add1/1 -> Sum2/2
  K1/1 -> Sum2/1

== system Receiver_UnderTest_Float/Receiver/Frame Recover/Frequency Recovery/Phase Shift FP ==
  In1 : Inport
  Phi : Inport  Port=2
  Complex Phase Shift : commutil2/Complex Phase Shift
      settings: SourceProductName=Communications System Toolbox  SourceProductBaseCode=CM
  Out1 : Outport
  wires:
  Phi/1 -> Complex Phase Shift/2
  In1/1 -> Complex Phase Shift/1
  Complex Phase Shift/1 -> Out1/1

== system Receiver_UnderTest_Float/Receiver/Gardner Timing Recovery/Gardner TED Blocks/Imag Error ==
  data : Inport
  strobe sum : Inport  Port=2
  Delay : Delay  DelayLength=1
  Product1 : Product
  Sub : Sum  Inputs=+-
  TED Buffer Update1 : Subsystem
  Out1 : Outport
  wires:
  TED Buffer Update1/1(Middle Indx) -> Product1/1
  Delay/1 -> TED Buffer Update1/1(new data)
  TED Buffer Update1/2(oldest) -> Sub/1
  strobe sum/1 -> TED Buffer Update1/2(strobe sum)
  data/1 -> Delay/1, Sub/2
  Sub/1 -> Product1/2
  Product1/1 -> Out1/1

== system Receiver_UnderTest_Float/Receiver/Gardner Timing Recovery/Gardner TED Blocks/Real Error ==
  data : Inport
  strobe sum : Inport  Port=2
  Delay : Delay  DelayLength=1
  Product1 : Product
  Sub : Sum  Inputs=+-
  TED Buffer Update1 : Subsystem
  Out1 : Outport
  wires:
  TED Buffer Update1/1(Middle Indx) -> Product1/1
  Delay/1 -> TED Buffer Update1/1(new data)
  TED Buffer Update1/2(oldest) -> Sub/1
  strobe sum/1 -> TED Buffer Update1/2(strobe sum)
  data/1 -> Delay/1, Sub/2
  Sub/1 -> Product1/2
  Product1/1 -> Out1/1

== system Receiver_UnderTest_Float/Receiver/Gardner Timing Recovery/InterpControl_Blocks1/Calculate New mu ==
  W : Inport
  NCOCounter : Inport  Port=2
  Math Reciprocal : Math  Operator=reciprocal  OutDataTypeStr=Inherit: Inherit via back propagation  RndMeth=Zero  SaturateOnIntegerOverflow=on
  Product : Product  OutDataTypeStr=Inherit: Inherit via back propagation
  mu : Outport
  wires:
  W/1 -> Math Reciprocal/1
  NCOCounter/1 -> Product/2
  Math Reciprocal/1 -> Product/1
  Product/1 -> mu/1

== system Receiver_UnderTest_Float/Receiver/Gardner Timing Recovery/InterpControl_Blocks1/Mod 1 ==
  In1 : Inport
  Add : Sum
  Compare To Constant : simulink/Logic and Bit Operations/Compare To Constant  relop=<  const=1  OutDataTypeStr=boolean
  Compare To Constant1 : simulink/Logic and Bit Operations/Compare To Constant  relop=>=  const=0  OutDataTypeStr=boolean
  Constant : Constant  OutDataTypeStr=fixdt(0,1,0)  SampleTime=-1
  Constant1 : Constant  OutDataTypeStr=fixdt(0,1,0)  SampleTime=-1
  Logical Operator : Logic  AllPortsSameDT=off  OutDataTypeStr=boolean
  Subtract : Sum  Inputs=+-
  Switch : Switch  Criteria=u2 > Threshold
  Switch1 : Switch
  Out1 : Outport
  wires:
  Logical Operator/1 -> Switch/2
  Compare To Constant/1 -> Logical Operator/2
  Compare To Constant1/1 -> Logical Operator/1
  In1/1 -> Subtract/1, Add/1, Switch/1, Compare To Constant/1, Compare To Constant1/1, Switch1/2
  Add/1 -> Switch1/3
  Subtract/1 -> Switch1/1
  Switch1/1 -> Switch/3
  Constant1/1 -> Add/2
  Constant/1 -> Subtract/2
  Switch/1 -> Out1/1

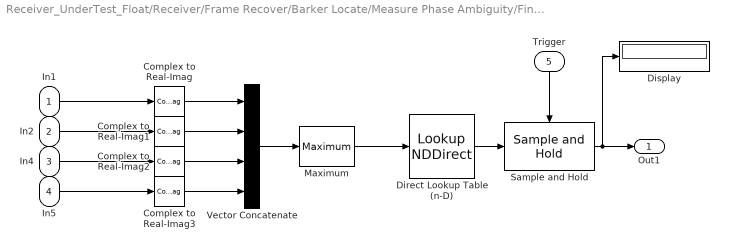
== system Receiver_UnderTest_Float/Receiver/Frame Recover/Barker Locate/Measure Phase Ambiguity/Find Max and Set Output Shift ==
  In1 : Inport
  In2 : Inport  Port=2
  In4 : Inport  Port=3
  In5 : Inport  Port=4
  Trigger : Inport  Port=5
  Complex to Real-Imag{,1..3} (4 alike) : ComplexToRealImag  Output=Imag
  Direct Lookup Table (n-D) : LookupNDDirect  NumberOfTableDimensions=1  Table=exp(-(0:pi/2:(pi*3/2)) .* 1i).'  DiagnosticForOutOfRangeInput=Error
  Display : Display
  Maximum : dspstat3/Maximum  operation=maximum  fcn=Index  indexBase=Zero  operateOver=Each column  Dimension=1  InputProcessing=Columns as channels (frame based)  reset=None  roiEnable=off  roiType=Rectangles  roiPortion=Entire ROI  roiOutput=Individual statistics for each ROI  roiFlag=off  roundingMode=Floor  overflowMode=off  accumDataTypeStr=Inherit: Same as product output  accumLastDataTypeStr=Inherit: Same as product output
  Sample and Hold : dspsigops/Sample and Hold  trig=Rising edge  initCond=1  latchinput=on
  Vector Concatenate : Concatenate  NumInputs=4
  Out1 : Outport
  wires:
  In4/1 -> Complex to Real-Imag2/1
  Vector Concatenate/1 -> Maximum/1
  In2/1 -> Complex to Real-Imag1/1
  Maximum/1 -> Direct Lookup Table (n-D)/1
  Complex to Real-Imag/1 -> Vector Concatenate/1
  Complex to Real-Imag3/1 -> Vector Concatenate/4
  In5/1 -> Complex to Real-Imag3/1
  Complex to Real-Imag1/1 -> Vector Concatenate/2
  Complex to Real-Imag2/1 -> Vector Concatenate/3
  Trigger/1 -> Sample and Hold/Trigger
  Sample and Hold/1 -> Display/1, Out1/1
  In1/1 -> Complex to Real-Imag/1
  Direct Lookup Table (n-D)/1 -> Sample and Hold/1

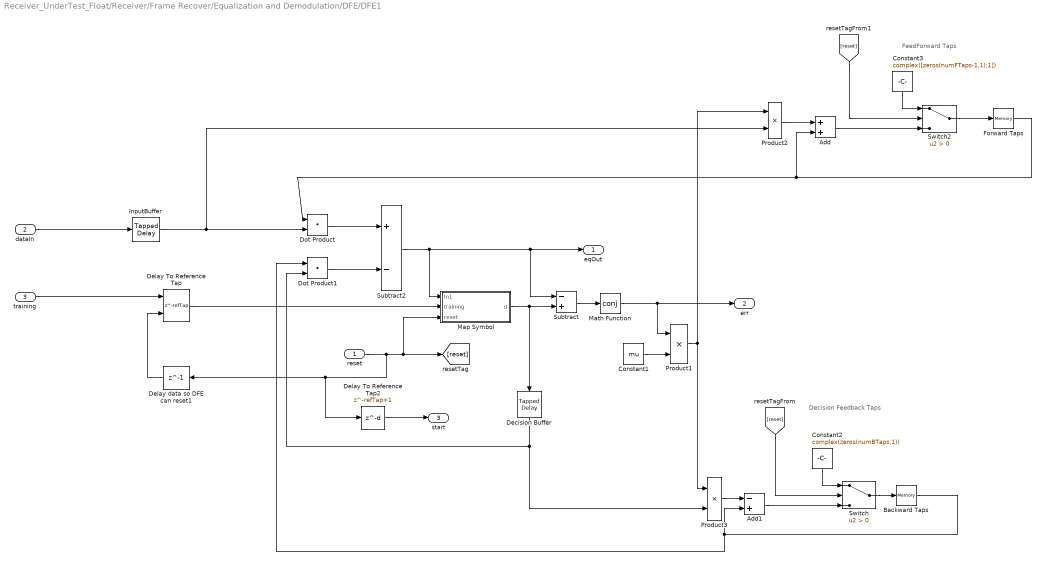
== system Receiver_UnderTest_Float/Receiver/Frame Recover/Equalization and Demodulation/DFE/DFE1 ==
  note: Decision Feedback Taps
  note: FeedForward Taps
  reset : Inport
  dataIn : Inport  Port=2
  training : Inport  Port=3
  Add : Sum
  Add1 : Sum  Inputs=-+
  Backward Taps : Memory  InitialCondition=complex(zeros(numBTaps,1))  InheritSampleTime=on
  Constant1 : Constant  Value=mu  SampleTime=-1
  Constant2 : Constant  Value=complex(zeros(numBTaps,1))  SampleTime=-1
  Constant3 : Constant  Value=complex([zeros(numFTaps-1,1);1])  SampleTime=-1
  Decision Buffer : simulink/Discrete/Tapped Delay  vinit=0.0  samptime=-1  NumDelays=numBTaps  DelayOrder=Oldest  includeCurrent=off
  Delay To Reference Tap : Delay  DelayLength=refTap  ExternalReset=Level
      settings: InputPortMap=u0,r5
  Delay To Reference Tap2 : Delay  DelayLength=refTap+1
  Delay data so DFE can reset1 : Delay  DelayLength=1
  Dot Product : DotProduct  SaturateOnIntegerOverflow=on  InputSameDT=on  OutDataTypeStr=Inherit: Inherit via internal rule
  Dot Product1 : DotProduct  SaturateOnIntegerOverflow=on  InputSameDT=on  OutDataTypeStr=Inherit: Inherit via internal rule
  Forward Taps : Memory  InitialCondition=[complex(zeros(numFTaps-1,1));1]  InheritSampleTime=on
  InputBuffer : simulink/Discrete/Tapped Delay  vinit=0.0  samptime=-1  NumDelays=numFTaps  DelayOrder=Oldest  includeCurrent=off
  Map Symbol : Subsystem
  Math Function : Math  Operator=conj  RndMeth=Zero  SaturateOnIntegerOverflow=on
  Product1 : Product
  Product2 : Product
  Product3 : Product
  Subtract : Sum  Inputs=-+
  Subtract2 : Sum  Inputs=+-
  Switch : Switch  Criteria=u2 > Threshold
  Switch2 : Switch  Criteria=u2 > Threshold
  eqOut : Outport
  err : Outport  Port=2
  start : Outport  Port=3
  wires:
  Delay To Reference Tap2/1 -> start/1
  Delay data so DFE can reset1/1 -> Delay To Reference Tap/2
  Delay To Reference Tap/1 -> Map Symbol/2(training)
  training/1 -> Delay To Reference Tap/1
  dataIn/1 -> InputBuffer/1
  Product3/1 -> Add1/1
  Product1/1 -> Product3/1, Product2/1
  Product2/1 -> Add/1
  [reset] -> Switch2/2
  Constant3/1 -> Switch2/1
  Add/1 -> Switch2/3
  Switch2/1 -> Forward Taps/1
  [reset] -> Switch/2
  Constant2/1 -> Switch/1
  Switch/1 -> Backward Taps/1
  Add1/1 -> Switch/3
  Decision Buffer/1 -> Dot Product1/2, Product3/2
  Backward Taps/1 -> Add1/2, Dot Product1/1
  Constant1/1 -> Product1/2
  reset/1 -> Map Symbol/3(reset), [reset], Delay data so DFE can reset1/1, Delay To Reference Tap2/1
  Map Symbol/1(d) -> Decision Buffer/1, Subtract/2
  Forward Taps/1 -> Add/2, Dot Product/1
  Math Function/1 -> Product1/1, err/1
  Subtract/1 -> Math Function/1
  Subtract2/1 -> eqOut/1, Subtract/1, Map Symbol/1(In1)
  Dot Product1/1 -> Subtract2/2
  Dot Product/1 -> Subtract2/1
  InputBuffer/1 -> Dot Product/2, Product2/2

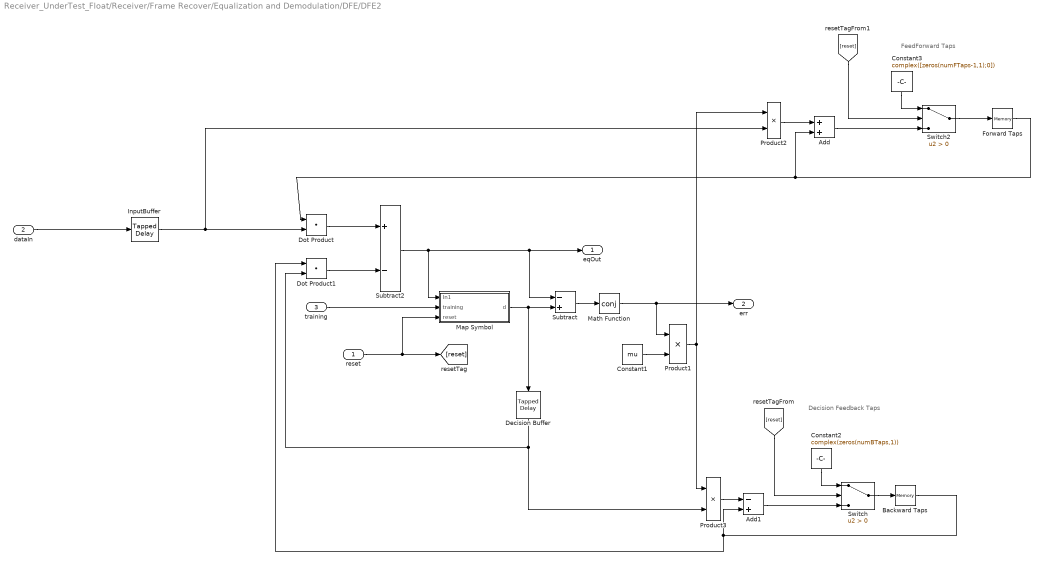
== system Receiver_UnderTest_Float/Receiver/Frame Recover/Equalization and Demodulation/DFE/DFE2 ==
  note: Decision Feedback Taps
  note: FeedForward Taps
  reset : Inport
  dataIn : Inport  Port=2  OutDataTypeStr=fixdt(1,16,15)  PortDimensions=1
  training : Inport  Port=3  OutDataTypeStr=fixdt(1,16,15)
  Add : Sum  OutDataTypeStr=fixdt(1,16,14)
  Add1 : Sum  Inputs=-+  OutDataTypeStr=fixdt(1,16,16)
  Backward Taps : Memory  InitialCondition=complex(zeros(numBTaps,1))  InheritSampleTime=on
  Constant1 : Constant  Value=mu  OutDataTypeStr=fixdt(0,16,22)  SampleTime=-1
  Constant2 : Constant  Value=complex(zeros(numBTaps,1))  OutDataTypeStr=fixdt(1,16,4)  SampleTime=-1
  Constant3 : Constant  Value=complex([zeros(numFTaps-1,1);0])  OutDataTypeStr=fixdt(1,16,4)  SampleTime=-1
  Decision Buffer : simulink/Discrete/Tapped Delay  vinit=0.0  samptime=-1  NumDelays=numBTaps  DelayOrder=Oldest  includeCurrent=off
  Dot Product : DotProduct  OutDataTypeStr=fixdt(1,16,16)  SaturateOnIntegerOverflow=on  InputSameDT=on
  Dot Product1 : DotProduct  OutDataTypeStr=fixdt(1,16,15)  SaturateOnIntegerOverflow=on  InputSameDT=on
  Forward Taps : Memory  InitialCondition=[complex(zeros(numFTaps-1,1));1]  InheritSampleTime=on
  InputBuffer : simulink/Discrete/Tapped Delay  vinit=0.0  samptime=-1  NumDelays=numFTaps  DelayOrder=Oldest  includeCurrent=off
  Map Symbol : Subsystem
  Math Function : Math  Operator=conj  RndMeth=Zero  SaturateOnIntegerOverflow=on
  Product1 : Product  OutDataTypeStr=fixdt(1,16,22)
  Product2 : Product  OutDataTypeStr=fixdt(1,16,23)
  Product3 : Product  OutDataTypeStr=fixdt(1,16,21)
  Subtract : Sum  Inputs=-+  OutDataTypeStr=fixdt(1,16,15)
  Subtract2 : Sum  Inputs=+-  OutDataTypeStr=fixdt(1,16,15)
  Switch : Switch  Criteria=u2 > Threshold  OutDataTypeStr=fixdt(1,16,15)
  Switch2 : Switch  Criteria=u2 > Threshold  OutDataTypeStr=fixdt(1,16,15)
  eqOut : Outport
  err : Outport  Port=2
  wires:
  training/1 -> Map Symbol/2(training)
  dataIn/1 -> InputBuffer/1
  Product3/1 -> Add1/1
  Product1/1 -> Product3/1, Product2/1
  Product2/1 -> Add/1
  [reset] -> Switch2/2
  Constant3/1 -> Switch2/1
  Add/1 -> Switch2/3
  Switch2/1 -> Forward Taps/1
  [reset] -> Switch/2
  Constant2/1 -> Switch/1
  Switch/1 -> Backward Taps/1
  Add1/1 -> Switch/3
  Decision Buffer/1 -> Dot Product1/2, Product3/2
  Backward Taps/1 -> Add1/2, Dot Product1/1
  Constant1/1 -> Product1/2
  reset/1 -> Map Symbol/3(reset), [reset]
  Map Symbol/1(d) -> Decision Buffer/1, Subtract/2
  Forward Taps/1 -> Add/2, Dot Product/1
  Math Function/1 -> Product1/1, err/1
  Subtract/1 -> Math Function/1
  Subtract2/1 -> eqOut/1, Subtract/1, Map Symbol/1(In1)
  Dot Product1/1 -> Subtract2/2
  Dot Product/1 -> Subtract2/1
  InputBuffer/1 -> Dot Product/2, Product2/2

== system Receiver_UnderTest_Float/Receiver/Frame Recover/Equalization and Demodulation/DFE/Packeted To Unpacked ==
  In1 : Inport
  Extract Bits : simulink/Logic and Bit Operations/Extract Bits  bitsToExtract=Range of bits  numBits=8  bitIdxRange=[1]  outScalingMode=Treat bit field as an integer
      settings: SourceProductName=Simulink
  Extract Bits1 : simulink/Logic and Bit Operations/Extract Bits  bitsToExtract=Range of bits  numBits=8  bitIdxRange=[0]  outScalingMode=Treat bit field as an integer
      settings: SourceProductName=Simulink
  Vector Concatenate : Concatenate
  Out1 : Outport
  wires:
  Vector Concatenate/1 -> Out1/1
  Extract Bits1/1 -> Vector Concatenate/2
  Extract Bits/1 -> Vector Concatenate/1
  In1/1 -> Extract Bits/1, Extract Bits1/1

== system Receiver_UnderTest_Float/Receiver/Gardner Timing Recovery/Gardner TED Blocks/Imag Error/TED Buffer Update1 ==
  new data : Inport
  strobe sum : Inport  Port=2
  Delay{,1..3} (4 alike) : Delay  DelayLength=1
  Multiport Switch{,1..3} (4 alike) : MultiPortSwitch  DataPortOrder=Zero-based contiguous  DataPortIndices={0,1,[2,3]}
  Zero bit : Constant  Value=0  SampleTime=1/RadioSampleRate
  Middle Indx : Outport
  oldest : Outport  Port=2
  wires:
  Multiport Switch/1 -> oldest/1, Delay/1
  Multiport Switch3/1 -> Delay3/1
  Multiport Switch2/1 -> Delay2/1, Middle Indx/1
  Multiport Switch1/1 -> Delay1/1
  Delay3/1 -> Multiport Switch3/2, Multiport Switch2/3, Multiport Switch1/4
  Zero bit/1 -> Multiport Switch2/4
  new data/1 -> Multiport Switch3/3, Multiport Switch3/4
  Delay2/1 -> Multiport Switch2/2, Multiport Switch1/3, Multiport Switch/4
  Delay1/1 -> Multiport Switch1/2, Multiport Switch/3
  Delay/1 -> Multiport Switch/2
  strobe sum/1 -> Multiport Switch/1, Multiport Switch1/1, Multiport Switch2/1, Multiport Switch3/1

== system Receiver_UnderTest_Float/Receiver/Gardner Timing Recovery/Gardner TED Blocks/Real Error/TED Buffer Update1 ==
  new data : Inport
  strobe sum : Inport  Port=2
  Delay{,1..3} (4 alike) : Delay  DelayLength=1
  Multiport Switch{,1..3} (4 alike) : MultiPortSwitch  DataPortOrder=Zero-based contiguous  DataPortIndices={0,1,[2,3]}
  Zero bit : Constant  Value=0  SampleTime=1/RadioSampleRate
  Middle Indx : Outport
  oldest : Outport  Port=2
  wires:
  Multiport Switch/1 -> oldest/1, Delay/1
  Multiport Switch3/1 -> Delay3/1
  Multiport Switch2/1 -> Delay2/1, Middle Indx/1
  Multiport Switch1/1 -> Delay1/1
  Delay3/1 -> Multiport Switch3/2, Multiport Switch2/3, Multiport Switch1/4
  Zero bit/1 -> Multiport Switch2/4
  new data/1 -> Multiport Switch3/3, Multiport Switch3/4
  Delay2/1 -> Multiport Switch2/2, Multiport Switch1/3, Multiport Switch/4
  Delay1/1 -> Multiport Switch1/2, Multiport Switch/3
  Delay/1 -> Multiport Switch/2
  strobe sum/1 -> Multiport Switch/1, Multiport Switch1/1, Multiport Switch2/1, Multiport Switch3/1

== system Receiver_UnderTest_Float/Receiver/Frame Recover/Equalization and Demodulation/DFE/DFE1/Map Symbol ==
  In1 : Inport
  training : Inport  Port=2
  reset : Inport  Port=3
  Decision Directed : Subsystem
  Delay : Delay  DelayLength=1
  HDL Counter : hdlsllib/Sources/HDL Counter  CountType=Count limited  CountInit=0  CountStep=1  CountMax=2^18  CountFromType=Initial value  CountFrom=0  CountResetPort=on  CountLoadPort=off  CountEnbPort=off  CountDirPort=off  CountDataType=Unsigned  CountWordLen=32  CountFracLen=0  CountSampTime=1
      settings: SourceProductBaseCode=HD
  Switch : Switch  Criteria=u2 > Threshold  Threshold=numTrainingSamples
  d : Outport
  wires:
  Delay/1 -> Switch/3
  training/1 -> Delay/1
  Decision Directed/1(decision) -> Switch/1
  HDL Counter/1 -> Switch/2
  reset/1 -> HDL Counter/1
  Switch/1 -> d/1
  In1/1 -> Decision Directed/1(eqOut)

== system Receiver_UnderTest_Float/Receiver/Frame Recover/Equalization and Demodulation/DFE/DFE2/Map Symbol ==
  In1 : Inport  OutDataTypeStr=fixdt(1,16,15)
  training : Inport  Port=2  OutDataTypeStr=fixdt(1,16,15)
  reset : Inport  Port=3
  Decision Directed : Subsystem
  Delay : Delay  DelayLength=1
  HDL Counter : hdlsllib/HDL Operations/HDL Counter  CountType=Count limited  CountInit=0  CountStep=1  CountMax=2^18  CountFromType=Initial value  CountFrom=0  CountResetPort=on  CountLoadPort=off  CountEnbPort=off  CountDirPort=off  CountDataType=Unsigned  CountWordLen=32  CountFracLen=0  CountSampTime=1
      settings: SourceProductName=HDL Coder  SourceProductBaseCode=HD
  Switch : Switch  Criteria=u2 > Threshold  Threshold=numTrainingSamples  OutDataTypeStr=fixdt(1,16,15)
  d : Outport
  wires:
  Delay/1 -> Switch/3
  training/1 -> Delay/1
  Decision Directed/1(decision) -> Switch/1
  HDL Counter/1 -> Switch/2
  reset/1 -> HDL Counter/1
  Switch/1 -> d/1
  In1/1 -> Decision Directed/1(eqOut)

== system Receiver_UnderTest_Float/Receiver/Frame Recover/Equalization and Demodulation/DFE/DFE1/Map Symbol/Decision Directed ==
  eqOut : Inport
  Compare To Zero : simulink/Logic and Bit Operations/Compare To Zero  relop=>=  OutDataTypeStr=boolean
  Compare To Zero1 : simulink/Logic and Bit Operations/Compare To Zero  relop=>=  OutDataTypeStr=boolean
  Complex to Real-Imag : ComplexToRealImag
  QPSK Decisions : LookupNDDirect  Table=[-0.7071 - 0.7071i, -0.7071 + 0.7071i; 0.7071 - 0.7071i, 0.7071 + 0.7071i]  DiagnosticForOutOfRangeInput=Error
  decision : Outport
  wires:
  QPSK Decisions/1 -> decision/1
  Compare To Zero1/1 -> QPSK Decisions/2
  Compare To Zero/1 -> QPSK Decisions/1
  Complex to Real-Imag/2 -> Compare To Zero1/1
  Complex to Real-Imag/1 -> Compare To Zero/1
  eqOut/1 -> Complex to Real-Imag/1

== system Receiver_UnderTest_Float/Receiver/Frame Recover/Equalization and Demodulation/DFE/DFE2/Map Symbol/Decision Directed ==
  eqOut : Inport  OutDataTypeStr=fixdt(1,16,15)
  Compare To Zero : simulink/Logic and Bit Operations/Compare To Zero  relop=>=  OutDataTypeStr=boolean
  Compare To Zero1 : simulink/Logic and Bit Operations/Compare To Zero  relop=>=  OutDataTypeStr=boolean
  Complex to Real-Imag : ComplexToRealImag
  QPSK Decisions : LookupNDDirect  Table=[-0.7071 - 0.7071i, -0.7071 + 0.7071i; 0.7071 - 0.7071i, 0.7071 + 0.7071i]  DiagnosticForOutOfRangeInput=Error
  decision : Outport
  wires:
  QPSK Decisions/1 -> decision/1
  Compare To Zero1/1 -> QPSK Decisions/2
  Compare To Zero/1 -> QPSK Decisions/1
  Complex to Real-Imag/2 -> Compare To Zero1/1
  Complex to Real-Imag/1 -> Compare To Zero/1
  eqOut/1 -> Complex to Real-Imag/1

== matlab function Receiver_UnderTest_Float/Receiver/CRC Check and DMA Pack/CRC Check ES/Debug CRC input ==
  data: u input; enable input; endFlag input; startFlag input
function fcn(u, enable,endFlag,startFlag)

persistent buffer crc count

if isempty(buffer)
   buffer = false(1700,1); 
    crc = comm.CRCDetector('Polynomial','z^32 + z^26 + z^23 + z^22 + z^16 + z^12 + z^11 + z^10 + z^8 + z^7 + z^5 + z^4 + z^2 + z + 1');
    count = 1;
end

if enable
    %buffer = [buffer(2:end);u];
    if startFlag
        count = 1;
    elseif count>1700-1
        count = 1;
    else
        count = count + 1;
    end
    buffer(count) = u;
    
    if endFlag
        disp(count)
        k = buffer(1:1632);
        [~,e] = crc(k);
        if e
            disp('Error');
        else
            disp('Pass');
        end
    end
    
end

== matlab function Receiver_UnderTest_Float/Receiver/Frame Recover/Enable Equalizer and Packet Decode (Latch) ==
  data: start input; enable output; validIn input
function enable = Counter(start,validIn)

persistent count maxCount lastEOF

if isempty(count)
    count = 0;
    maxCount = 2^16; % Largest possible packet length
    lastEOF = false;
end

eof = false;

if validIn
    % Got a barker preamble start allowing data into equalizer
    if start
        count = maxCount;
    end
    
    % Check on change from true to false
    if lastEOF && ~eof
        %     fprintf('Frame end reached\n');
        count = 0;
    end
    lastEOF = eof;
    
    % Past end of max frame size
    if count>0
        count = count - 1;
    end
    
    % Enable downstream
    enable = count>0;
else
    enable = false;
end

== matlab function Receiver_UnderTest_Float/Check Receiver/DMA Capture ==
  data: bytes input; validOut input; sync input; payloadLen input
function fcn(bytes, validOut, sync, payloadLen)

persistent frameBuffer byteCounter fullPayloadBits

if isempty(frameBuffer)
    frameBuffer = false(2^16,1);
    byteCounter = 0;
    fullPayloadBits = uint16(0);
end

if validOut
    if sync
        byteCounter = 32;
        frameBuffer(1:byteCounter) = bitget(bytes,1:32);
        fullPayloadBits = uint16(payloadLen*8);
        
    elseif byteCounter<fullPayloadBits
        frameBuffer(byteCounter+1:byteCounter+32) = bitget(bytes,1:32);
        byteCounter = byteCounter + 32;
    else
        if bytes>0
            disp('CRC Error (Outside)');
        else
            disp('Frame passed CRC (Outside)');
        end
    end
end

== matlab function Receiver_UnderTest_Float/Receiver/CRC Check and DMA Pack/CRC Check ES/Check CRC Result (DEBUG) ==
  data: bits input; start input; done input; valid input; err input
function fcn(bits, start, done, valid, err)

persistent buffer

if isempty(buffer)
    buffer = fi(false(1032,1),0,1,0);
end

buffer = [buffer(2:end);bits];

if done && valid
    if err
        fprintf('CRC Error (HDL CRC)\n');
    else
        fprintf('CRC Passed (HDL CRC)\n');
    end
end
if err % Flag if any error every occurs, if it occurs alone it means given crc is not long enough
    fprintf('CRC Error Type 2 (HDL CRC)\n');
end
